simulink model "Loops4"  (Simulink 8.7)
settings: Solver=ode45  StartTime=0.0  StopTime=10.0  RelTol=1e-3
settings Model: Creator=scaife  LastModifiedBy=bourbouh  ExtModeAutoUpdateStatusClock=off
settings DataIOCC: SignalLoggingSaveFormat=ModelDataLogs  SignalLoggingName=sigsOut
settings OptimizationCC: InitFltsAndDblsToZero=on
settings DebuggingCC: SaveWithParameterizedLinksMsg=none  SignalResolutionControl=TryResolveAllWithWarning  MultiTaskDSMMsg=warning  MultiTaskCondExecSysMsg=none
settings HardwareCC: TargetUnknown=on
settings SFSimCC: SimParseCustomCode=off
settings GRTTargetCC: TargetFcnLib=ansi_tfl_tmw.mat  ModelReferenceCompliant=off  GeneratePreprocessorConditionals=Use local settings  CombineOutputUpdateFcns=off  MatFileLogging=off  GRTInterface=on

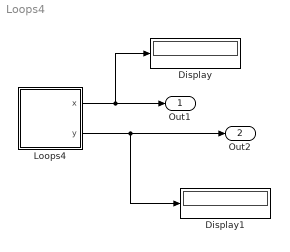
== system Loops4 ==
  Display : Display
  Display1 : Display
  Loops4 : Stateflow chart  TreatAsAtomicUnit=on
  Out1 : Outport
  Out2 : Outport  Port=2
  wires:
  Loops4/1(x) -> Out1/1, Display/1
  Loops4/2(y) -> Out2/1, Display1/1

== stateflow chart Loops4 ==
  state A
  state B
  B -> A : {y=!y}
  (default) -> A
  A -> (junction 7) : {x=0;}
  (junction 7) -> (junction 8) [order 2] : [!y]
  (junction 7) -> (junction 9) [order 1] : [y]
  (junction 9) -> (junction 9) [order 1] : [x<5]
      | {x++;}
  (junction 8) -> (junction 8) [order 1] : [x<10]
      | {x++;}
  (junction 8) -> B [order 2]
  (junction 9) -> B [order 2]
  data: x output int32; y output boolean
